simulink model "active_cruise_CTG"  (R2014a)
settings: Solver=ode45  StartTime=0.0  StopTime=10.0  RelTol=1e-3
settings Model: Creator=Ye  LastModifiedBy=Ye

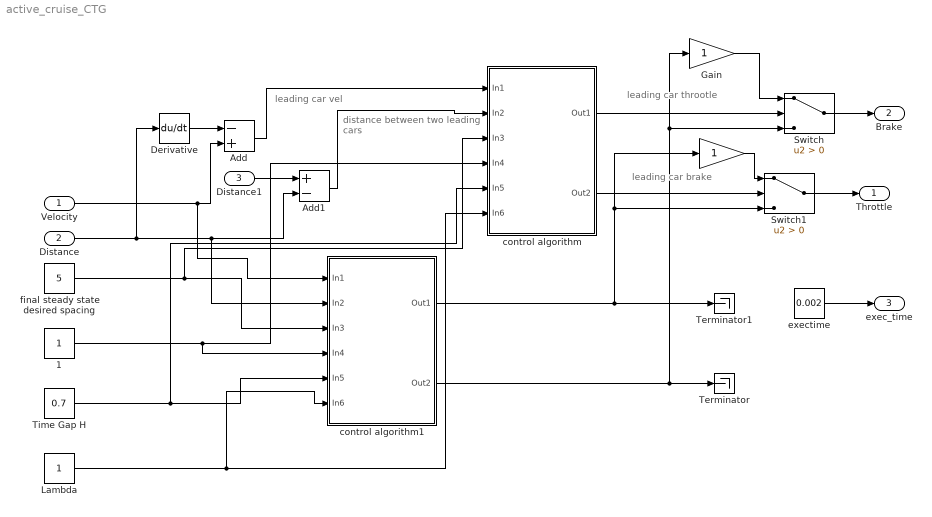
== system active_cruise_CTG ==
  note: leading car brake
  note: leading car throotle
  note: distance between two leading cars
  note: leading car vel
  Velocity : Inport
  Distance : Inport  Port=2
  Distance1 : Inport  Port=3
  " " : Gain
  1 : Constant
  Add : Sum  Inputs=-+
  Add1 : Sum  Inputs=+-
  Derivative : Derivative
  Gain : Gain
  Lambda : Constant
  Switch : Switch  Criteria=u2 > Threshold
  Switch1 : Switch  Criteria=u2 > Threshold
  Terminator : Terminator
  Terminator1 : Terminator
  Time Gap H : Constant  Value=0.7
  control algorithm : Subsystem
  control algorithm1 : Subsystem
  exectime : Constant  Value=0.002
  final steady state desired spacing : Constant  Value=5
  Throttle : Outport
  Brake : Outport  Port=2
  exec_time : Outport  Port=3
  wires:
  Velocity/1 -> Add/2, control algorithm1/1(In1)
  Distance/1 -> Derivative/1, Add1/2, control algorithm1/2(In2)
  final steady state desired spacing/1 -> control algorithm/3(In3), control algorithm1/3(In3)
  1/1 -> control algorithm/4(In4), control algorithm1/4(In4)
  Time Gap H/1 -> control algorithm/5(In5), control algorithm1/5(In5)
  Lambda/1 -> control algorithm/6(In6), control algorithm1/6(In6)
  control algorithm1/1(Out1) -> Terminator1/1, Switch1/3, " "/1
  control algorithm1/2(Out2) -> Terminator/1, Switch/3, Gain/1
  Derivative/1 -> Add/1
  Add/1 -> control algorithm/1(In1)
  Distance1/1 -> Add1/1
  Add1/1 -> control algorithm/2(In2)
  control algorithm/1(Out1) -> Switch/2
  control algorithm/2(Out2) -> Switch1/2
  Switch/1 -> Brake/1
  Gain/1 -> Switch/1
  " "/1 -> Switch1/1
  Switch1/1 -> Throttle/1
  exectime/1 -> exec_time/1

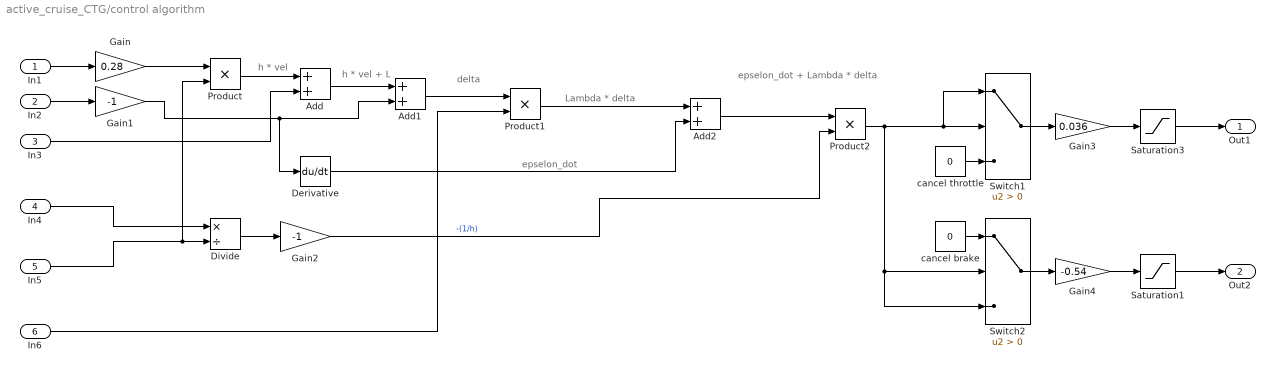
== system active_cruise_CTG/control algorithm ==
  note: Lambda * delta
  note: delta
  note: h * vel
  note: h * vel + L
  note: epselon_dot + Lambda * delta
  note: epselon_dot
  In1 : Inport
  In2 : Inport  Port=2
  In3 : Inport  Port=3
  In4 : Inport  Port=4
  In5 : Inport  Port=5
  In6 : Inport  Port=6
  Add : Sum
  Add1 : Sum
  Add2 : Sum
  Derivative : Derivative
  Divide : Product  Inputs=*/
  Gain : Gain  Gain=0.28
  Gain1 : Gain  Gain=-1
  Gain2 : Gain  Gain=-1
  Gain3 : Gain  Gain=0.036
  Gain4 : Gain  Gain=-0.54
  Product : Product
  Product1 : Product
  Product2 : Product
  Saturation1 : Saturate  UpperLimit=15  LowerLimit=0
  Saturation3 : Saturate  UpperLimit=1  LowerLimit=0
  Switch1 : Switch  Criteria=u2 > Threshold  SaturateOnIntegerOverflow=on
  Switch2 : Switch  Criteria=u2 > Threshold  SaturateOnIntegerOverflow=on
  cancel brake : Constant  Value=0
  cancel throttle : Constant  Value=0
  Out1 : Outport
  Out2 : Outport  Port=2
  wires:
  Gain4/1 -> Saturation1/1
  Switch2/1 -> Gain4/1
  Saturation1/1 -> Out2/1
  Gain2/1 -> Product2/2  "-(1/h)"
  In6/1 -> Product1/2
  Gain3/1 -> Saturation3/1
  cancel brake/1 -> Switch2/1
  Add/1 -> Add1/1
  cancel throttle/1 -> Switch1/3
  Gain1/1 -> Add1/2, Derivative/1
  Divide/1 -> Gain2/1
  Derivative/1 -> Add2/2
  Add1/1 -> Product1/1
  Product1/1 -> Add2/1
  Saturation3/1 -> Out1/1
  In2/1 -> Gain1/1
  Add2/1 -> Product2/1
  Switch1/1 -> Gain3/1
  Product2/1 -> Switch1/2, Switch1/1, Switch2/3, Switch2/2
  Gain/1 -> Product/1
  In3/1 -> Add/2
  Product/1 -> Add/1
  In1/1 -> Gain/1
  In5/1 -> Divide/2, Product/2
  In4/1 -> Divide/1

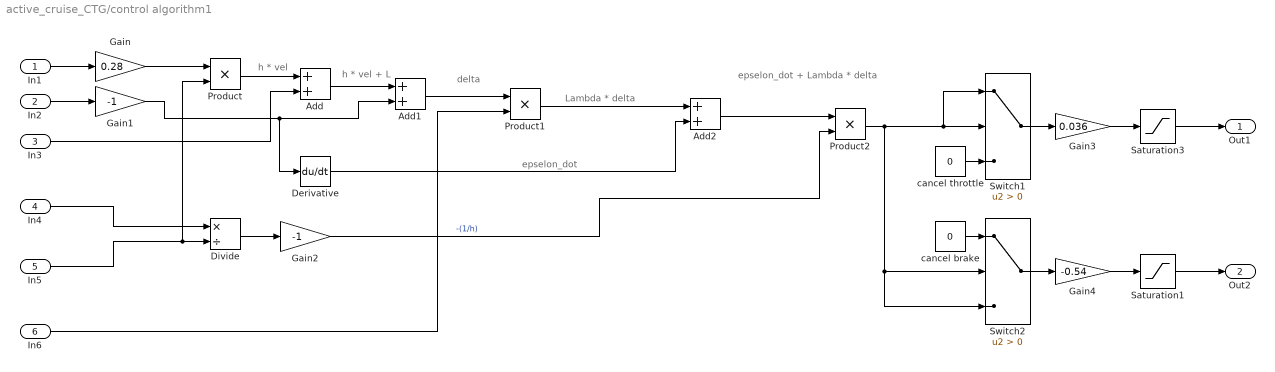
== system active_cruise_CTG/control algorithm1 ==
  note: epselon_dot
  note: epselon_dot + Lambda * delta
  note: h * vel + L
  note: h * vel
  note: delta
  note: Lambda * delta
  In1 : Inport
  In2 : Inport  Port=2
  In3 : Inport  Port=3
  In4 : Inport  Port=4
  In5 : Inport  Port=5
  In6 : Inport  Port=6
  Add : Sum
  Add1 : Sum
  Add2 : Sum
  Derivative : Derivative
  Divide : Product  Inputs=*/
  Gain : Gain  Gain=0.28
  Gain1 : Gain  Gain=-1
  Gain2 : Gain  Gain=-1
  Gain3 : Gain  Gain=0.036
  Gain4 : Gain  Gain=-0.54
  Product : Product
  Product1 : Product
  Product2 : Product
  Saturation1 : Saturate  UpperLimit=15  LowerLimit=0
  Saturation3 : Saturate  UpperLimit=1  LowerLimit=0
  Switch1 : Switch  Criteria=u2 > Threshold  SaturateOnIntegerOverflow=on
  Switch2 : Switch  Criteria=u2 > Threshold  SaturateOnIntegerOverflow=on
  cancel brake : Constant  Value=0
  cancel throttle : Constant  Value=0
  Out1 : Outport
  Out2 : Outport  Port=2
  wires:
  In4/1 -> Divide/1
  In5/1 -> Product/2, Divide/2
  In1/1 -> Gain/1
  Product/1 -> Add/1
  In3/1 -> Add/2
  Gain/1 -> Product/1
  Product2/1 -> Switch2/2, Switch2/3, Switch1/1, Switch1/2
  Switch1/1 -> Gain3/1
  Add2/1 -> Product2/1
  In2/1 -> Gain1/1
  Saturation3/1 -> Out1/1
  Product1/1 -> Add2/1
  Add1/1 -> Product1/1
  Derivative/1 -> Add2/2
  Divide/1 -> Gain2/1
  Gain1/1 -> Derivative/1, Add1/2
  cancel throttle/1 -> Switch1/3
  Add/1 -> Add1/1
  cancel brake/1 -> Switch2/1
  Gain3/1 -> Saturation3/1
  In6/1 -> Product1/2
  Gain2/1 -> Product2/2  "-(1/h)"
  Saturation1/1 -> Out2/1
  Switch2/1 -> Gain4/1
  Gain4/1 -> Saturation1/1
